simulink model "operation_ex"  (R2018a)
settings: Solver=VariableStepAuto  StartTime=0.0  StopTime=10.0  RelTol=1e-3
settings Model: Creator=lenovo  LastModifiedBy=DELL

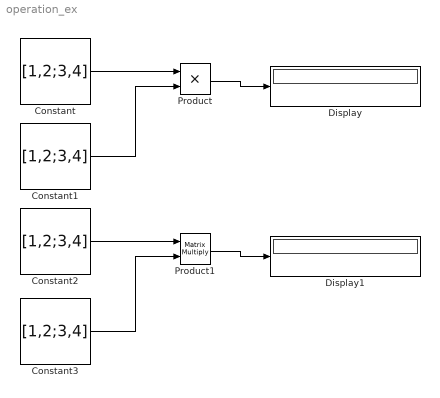
== system operation_ex ==
  Constant{,1..3} (4 alike) : Constant  Value=[1,2;3,4]
  Display : Display
  Display1 : Display
  Product : Product
  Product1 : Product  Multiplication=Matrix(*)
  wires:
  Constant/1 -> Product/1
  Constant2/1 -> Product1/1
  Constant3/1 -> Product1/2
  Constant1/1 -> Product/2
  Product/1 -> Display/1
  Product1/1 -> Display1/1
